simulink model "sampleModel7323_pp_1_1"  (R2018a)
settings: Solver=VariableStepAuto  StartTime=0.0  StopTime=10.0  RelTol=1e-3
undefined symbols (not defined in the file): DiscIntNeverNeededParam
libraries: simulink x65
(part 1 of 2)
settings Model: Creator=cyfuzz  LastModifiedBy=shafiul
settings CodeAppCC: StateflowObjectComments=on

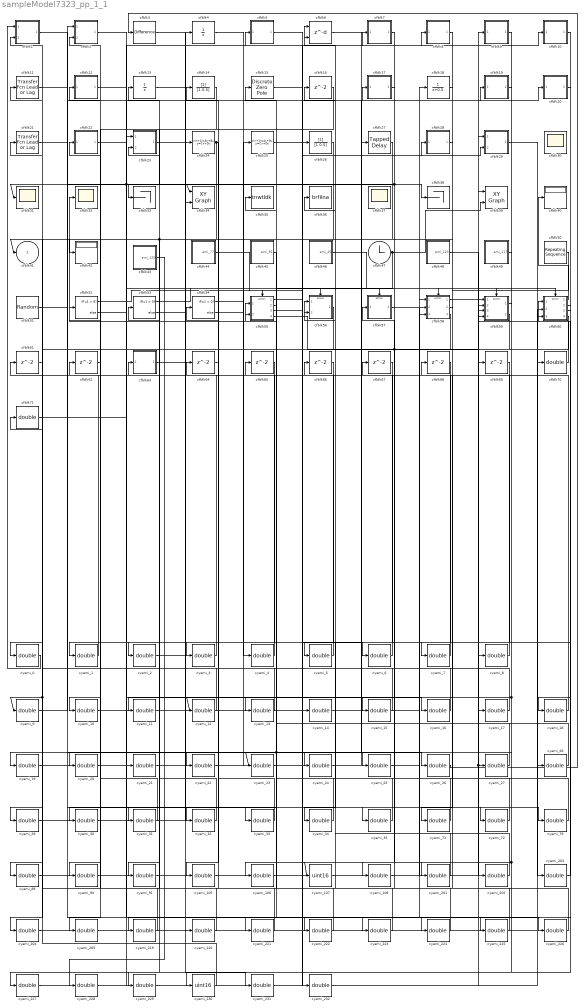
== system sampleModel7323_pp_1_1 ==
  cfblk1 : Subsystem  TreatAsAtomicUnit=on
  cfblk10 : Subsystem  TreatAsAtomicUnit=on
  cfblk11 : simulink/Discrete/Transfer Fcn Lead or Lag  PoleZ=0.95  ZeroZ=0.75  ICPrevOutput=0.0  ICPrevInput=0.0  DoSatur=off
      settings: SourceProductName=Simulink  SourceProductBaseCode=SL
  cfblk12 : Subsystem  TreatAsAtomicUnit=on
  cfblk13 : UnitDelay
  cfblk14 : DiscreteFilter  SampleTime=1
  cfblk15 : DiscreteZeroPole  Poles=[0 0.5]  Gain=1
  cfblk{16,61..62,64..69} (9 alike) : Delay  SampleTime=1
  cfblk17 : Subsystem  TreatAsAtomicUnit=on
  cfblk18 : DiscreteTransferFcn  SampleTime=1
  cfblk19 : Subsystem  TreatAsAtomicUnit=on
  cfblk2 : Subsystem  TreatAsAtomicUnit=on
  cfblk20 : Subsystem  TreatAsAtomicUnit=on
  cfblk21 : simulink/Discrete/Transfer Fcn Lead or Lag  PoleZ=0.95  ZeroZ=0.75  ICPrevOutput=0.0  ICPrevInput=0.0  DoSatur=off
      settings: SourceProductName=Simulink  SourceProductBaseCode=SL
  cfblk22 : Subsystem  TreatAsAtomicUnit=on
  cfblk23 : Subsystem  TreatAsAtomicUnit=on
  cfblk24 : DiscreteStateSpace
  cfblk25 : DiscreteStateSpace
  cfblk26 : DiscreteFilter  SampleTime=1
  cfblk27 : simulink/Discrete/Tapped Delay  vinit=0.0  samptime=-1  NumDelays=1  DelayOrder=Oldest  includeCurrent=off
  cfblk28 : Subsystem  TreatAsAtomicUnit=on
  cfblk29 : Subsystem  TreatAsAtomicUnit=on
  cfblk3 : simulink/Discrete/Difference  ICPrevInput=0.0  OutMin=[]  OutMax=[]  OutDataTypeStr=double  OutputDataTypeScalingMode=double  OutDataType=fixdt(1, 16)  OutScaling=2^-10  DoSatur=off
  cfblk{30..32,37} (4 alike) : Scope
      cfblk30 settings: Floating=on
      cfblk37 settings: Floating=on
  cfblk33 : Terminator
  cfblk34 : simulink/Sinks/XY Graph  xmin=-1  xmax=1  ymin=-1  ymax=1  st=-1
  cfblk35 : ToWorkspace  VariableName=tnwtldk  SaveFormat=Timeseries  SampleTime=-1
  cfblk36 : ToWorkspace  VariableName=brfiina  SaveFormat=Timeseries  SampleTime=-1
  cfblk38 : Terminator
  cfblk39 : simulink/Sinks/XY Graph  xmin=-1  xmax=1  ymin=-1  ymax=1  st=-1
  cfblk4 : UnitDelay
  cfblk40 : Display
  cfblk42 : Display
  cfblk43 : Subsystem  TreatAsAtomicUnit=on
  cfblk44 : Subsystem  TreatAsAtomicUnit=on
  cfblk45 : Subsystem  TreatAsAtomicUnit=on
  cfblk46 : Subsystem  TreatAsAtomicUnit=on
  cfblk47 : Clock
  cfblk48 : Subsystem  TreatAsAtomicUnit=on
  cfblk49 : Subsystem  TreatAsAtomicUnit=on
  cfblk5 : Subsystem  TreatAsAtomicUnit=on
  cfblk50 : simulink/Sources/Repeating Sequence  rep_seq_t=[0 2]  rep_seq_y=[0 2]
  cfblk51 : UniformRandomNumber  SampleTime=0.1
  cfblk52 : If  SampleTime=1
  cfblk53 : If  SampleTime=1
  cfblk54 : If  SampleTime=1
  cfblk55 : Subsystem  TreatAsAtomicUnit=on
  cfblk56 : Subsystem  TreatAsAtomicUnit=on
  cfblk57 : Subsystem  TreatAsAtomicUnit=on
  cfblk58 : Subsystem  TreatAsAtomicUnit=on
  cfblk59 : Subsystem  TreatAsAtomicUnit=on
  cfblk6 : Delay  DelayLengthSource=Input port  SampleTime=1
      settings: InputPortMap=u0,p1
  cfblk60 : Subsystem  TreatAsAtomicUnit=on
  cfblk63 : Subsystem  TreatAsAtomicUnit=on
  cfblk7 : Subsystem  TreatAsAtomicUnit=on
  cfblk70 : DataTypeConversion  OutDataTypeStr=double
  cfblk71 : DataTypeConversion  OutDataTypeStr=double
  cfblk8 : Subsystem  TreatAsAtomicUnit=on
  cfblk9 : Subsystem  TreatAsAtomicUnit=on
  cyemi_{0..35,71..72,79,89..91,105..106,108,201..205,219..229,231..232} (63 alike) : DataTypeConversion  OutDataTypeStr=double
  cyemi_107 : DataTypeConversion  OutDataTypeStr=uint16
  cyemi_230 : DataTypeConversion  OutDataTypeStr=uint16
  cfblk41 : Outport
  wires:
  cfblk55/2(cfblk13) -> cfblk32/1
  cfblk24/1 -> cfblk41/1, cyemi_91/1, cyemi_32/1
  cfblk56/1(cfblk2) -> cyemi_9/1, cyemi_204/1
  cfblk60/1(cfblk2) -> cfblk40/1
  cfblk11/1 -> cfblk38/1
  cfblk16/1 -> cfblk33/1
  cfblk47/1 -> cfblk39/2, cyemi_13/1
  cfblk60/4(cfblk16) -> cyemi_108/1, cyemi_221/1
  cfblk52/1 -> cfblk55/Action
  cfblk52/2 -> cfblk56/Action
  cfblk53/1 -> cfblk57/Action
  cfblk53/2 -> cfblk58/Action
  cfblk54/1 -> cfblk59/Action
  cfblk54/2 -> cfblk60/Action
  cfblk70/1 -> cfblk39/1
  cfblk61/1 -> cyemi_0/1
  cfblk67/1 -> cyemi_1/1
  cfblk60/2(cfblk14) -> cyemi_2/1
  cyemi_3/1 -> cfblk11/1
  cfblk4/1 -> cyemi_4/1
  cyemi_5/1 -> cfblk13/1
  cfblk58/2(cfblk16) -> cyemi_5/1
  cyemi_6/1 -> cfblk14/1
  cyemi_7/1 -> cfblk15/1
  cfblk59/2(cfblk16) -> cyemi_7/1
  cyemi_8/1 -> cfblk16/1
  cfblk55/4(cfblk15) -> cyemi_8/1
  cyemi_10/1 -> cfblk18/1
  cfblk14/1 -> cyemi_10/1
  cfblk59/1(cfblk2) -> cyemi_11/1
  cfblk55/3(cfblk14) -> cyemi_14/1
  cyemi_15/1 -> cfblk21/1
  cfblk13/1 -> cyemi_16/1
  cfblk58/1(cfblk2) -> cyemi_17/1
  cfblk60/3(cfblk15) -> cyemi_18/1
  cyemi_19/1 -> cfblk24/1
  cfblk50/1 -> cyemi_19/1
  cyemi_20/1 -> cfblk25/1
  cyemi_21/1 -> cfblk26/1
  cfblk71/1 -> cyemi_21/1
  cyemi_22/1 -> cfblk27/1
  cfblk51/1 -> cyemi_24/1
  cyemi_26/1 -> cfblk3/1
  cfblk6/1 -> cyemi_26/1
  cyemi_27/1 -> cfblk35/1
  cyemi_28/1 -> cfblk36/1
  cyemi_29/1 -> cfblk4/1
  cfblk58/3(cfblk17) -> cyemi_29/1
  cyemi_31/1 -> cfblk52/1
  cfblk66/1 -> cyemi_31/1
  cyemi_32/1 -> cfblk53/1
  cyemi_33/1 -> cfblk54/1
  cfblk68/1 -> cyemi_33/1
  cyemi_34/1 -> cfblk55/1(cfblk1)
  cfblk69/1 -> cyemi_34/1
  cyemi_35/1 -> cfblk55/2(cfblk12)
  cyemi_71/1 -> cfblk56/1(cfblk1)
  cfblk18/1 -> cyemi_71/1
  cyemi_72/1 -> cfblk56/2(cfblk7)
  cyemi_79/1 -> cfblk57/1(cfblk1)
  cfblk55/1(cfblk2) -> cyemi_79/1
  cyemi_89/1 -> cfblk58/1(cfblk1)
  cfblk27/1 -> cyemi_89/1
  cyemi_90/1 -> cfblk58/2(cfblk14)
  cfblk65/1 -> cyemi_90/1
  cyemi_91/1 -> cfblk58/3(cfblk15)
  cyemi_105/1 -> cfblk59/1(cfblk1)
  cfblk64/1 -> cyemi_105/1
  cyemi_106/1 -> cfblk59/2(cfblk13)
  cyemi_107/1 -> cfblk59/3(cfblk14)
  cyemi_108/1 -> cfblk59/4(cfblk15)
  cyemi_201/1 -> cfblk6/1
  cyemi_202/1 -> cfblk6/2
  cyemi_203/1 -> cfblk60/1(cfblk1)
  cyemi_204/1 -> cfblk60/2(cfblk12)
  cyemi_205/1 -> cfblk60/3(cfblk13)
  cfblk62/1 -> cyemi_205/1
  cyemi_219/1 -> cfblk61/1
  cyemi_220/1 -> cfblk62/1
  cyemi_222/1 -> cfblk64/1
  cyemi_223/1 -> cfblk65/1
  cfblk25/1 -> cyemi_223/1
  cyemi_224/1 -> cfblk66/1
  cyemi_225/1 -> cfblk67/1
  cfblk21/1 -> cyemi_225/1
  cyemi_226/1 -> cfblk68/1
  cfblk57/1(cfblk2) -> cyemi_226/1
  cyemi_227/1 -> cfblk69/1
  cyemi_229/1 -> cfblk70/1
  cfblk26/1 -> cyemi_229/1
  cyemi_230/1 -> cfblk71/1
  cfblk3/1 -> cyemi_231/1
  cfblk15/1 -> cyemi_232/1
  cyemi_221/1 -> cfblk63/1(emi_6)
  cfblk63/1(emi_7) -> cyemi_35/1
  cyemi_11/1 -> cfblk19/1(emi_9)
  cfblk19/1(emi_10) -> cyemi_201/1
  cyemi_228/1 -> cfblk7/1(emi_15)
  cfblk7/1(emi_16) -> cyemi_106/1, cfblk31/1
  cyemi_9/1 -> cfblk17/1(emi_30)
  cfblk17/1(emi_31) -> cyemi_22/1, cfblk34/1
  cyemi_4/1 -> cfblk12/1(emi_39)
  cfblk12/1(emi_40) -> cyemi_15/1
  cfblk46/1(emi_45) -> cyemi_28/1
  cyemi_24/1 -> cfblk29/1(emi_47)
  cyemi_25/1 -> cfblk29/2(emi_48)
  cfblk29/1(emi_49) -> cyemi_203/1
  cyemi_16/1 -> cfblk22/1(emi_54)
  cfblk22/1(emi_55) -> cyemi_224/1, cfblk34/2
  cyemi_23/1 -> cfblk28/1(emi_64)
  cfblk28/1(emi_65) -> cyemi_3/1
  cyemi_14/1 -> cfblk20/1(emi_67)
  cfblk20/1(emi_68) -> cyemi_227/1
  cyemi_17/1 -> cfblk23/1(emi_73)
  cyemi_18/1 -> cfblk23/2(emi_74)
  cfblk23/1(emi_75) -> cyemi_220/1
  cfblk44/1(emi_77) -> cyemi_6/1
  cyemi_30/1 -> cfblk5/1(emi_79)
  cfblk5/1(emi_80) -> cyemi_25/1
  cyemi_2/1 -> cfblk10/1(emi_82)
  cfblk10/1(emi_83) -> cyemi_219/1
  cyemi_231/1 -> cfblk8/1(emi_85)
  cfblk8/1(emi_86) -> cfblk42/1
  cfblk45/1(emi_91) -> cyemi_30/1, cyemi_23/1
  cyemi_12/1 -> cfblk2/1(emi_103)
  cyemi_13/1 -> cfblk2/2(emi_104)
  cfblk2/1(emi_105) -> cyemi_222/1
  cyemi_232/1 -> cfblk9/1(emi_107)
  cfblk9/1(emi_108) -> cyemi_20/1, cyemi_12/1
  cyemi_0/1 -> cfblk1/1(emi_113)
  cyemi_1/1 -> cfblk1/2(emi_114)
  cfblk1/1(emi_115) -> cyemi_72/1
  cfblk49/1(emi_117) -> cyemi_107/1, cyemi_230/1
  cfblk48/1(emi_123) -> cyemi_202/1, cyemi_27/1
  cfblk43/1(emi_125) -> cyemi_228/1

== system sampleModel7323_pp_1_1/cfblk1 ==
  emi_113 : Inport  Partition=on  PartitionDimension=1  PartitionWidth=1  PartitionOffset=0
  emi_114 : Inport  Port=2  Partition=on  PartitionDimension=1  PartitionWidth=1  PartitionOffset=0
  For Each : ForEach  DisableCoverage=on  IndexMode=One-based
  cfblk1 : Delay  ShowEnablePort=on  SampleTime=1
      settings: InputPortMap=u0,e6
  emi_115 : Outport  ConcatenationDimension=1
  wires:
  emi_113/1 -> cfblk1/1
  emi_114/1 -> cfblk1/2
  cfblk1/1 -> emi_115/1

== system sampleModel7323_pp_1_1/cfblk10 ==
  emi_82 : Inport  Partition=on  PartitionDimension=1  PartitionWidth=1  PartitionOffset=0
  For Each : ForEach  DisableCoverage=on  IndexMode=One-based
  cfblk10 : simulink/Discrete/Difference  ICPrevInput=0.0  OutMin=[]  OutMax=[]  OutDataTypeStr=double  OutputDataTypeScalingMode=double  OutDataType=fixdt(1, 16)  OutScaling=2^-10  DoSatur=off
  emi_83 : Outport  ConcatenationDimension=1
  wires:
  emi_82/1 -> cfblk10/1
  cfblk10/1 -> emi_83/1

== system sampleModel7323_pp_1_1/cfblk12 ==
  emi_39 : Inport  Partition=on  PartitionDimension=1  PartitionWidth=1  PartitionOffset=0
  For Each : ForEach  DisableCoverage=on  IndexMode=One-based
  cfblk12 : DiscreteFilter  SampleTime=1
  emi_40 : Outport  ConcatenationDimension=1
  wires:
  emi_39/1 -> cfblk12/1
  cfblk12/1 -> emi_40/1

== system sampleModel7323_pp_1_1/cfblk17 ==
  emi_30 : Inport  Partition=on  PartitionDimension=1  PartitionWidth=1  PartitionOffset=0
  For Each : ForEach  DisableCoverage=on  IndexMode=One-based
  cfblk17 : simulink/Discrete/Tapped Delay  vinit=0.0  samptime=-1  NumDelays=1  DelayOrder=Oldest  includeCurrent=off
  emi_31 : Outport  ConcatenationDimension=1
  wires:
  emi_30/1 -> cfblk17/1
  cfblk17/1 -> emi_31/1

== system sampleModel7323_pp_1_1/cfblk19 ==
  emi_9 : Inport  Partition=on  PartitionDimension=1  PartitionWidth=1  PartitionOffset=0
  For Each : ForEach  DisableCoverage=on  IndexMode=One-based
  cfblk19 : simulink/Discrete/Difference  ICPrevInput=0.0  OutMin=[]  OutMax=[]  OutDataTypeStr=double  OutputDataTypeScalingMode=double  OutDataType=fixdt(1, 16)  OutScaling=2^-10  DoSatur=off
  emi_10 : Outport  ConcatenationDimension=1
  wires:
  emi_9/1 -> cfblk19/1
  cfblk19/1 -> emi_10/1

== system sampleModel7323_pp_1_1/cfblk2 ==
  emi_103 : Inport  Partition=on  PartitionDimension=1  PartitionWidth=1  PartitionOffset=0
  emi_104 : Inport  Port=2  Partition=on  PartitionDimension=1  PartitionWidth=1  PartitionOffset=0
  For Each : ForEach  DisableCoverage=on  IndexMode=One-based
  cfblk2 : Delay  ShowEnablePort=on  SampleTime=1
      settings: InputPortMap=u0,e6
  emi_105 : Outport  ConcatenationDimension=1
  wires:
  emi_103/1 -> cfblk2/1
  emi_104/1 -> cfblk2/2
  cfblk2/1 -> emi_105/1

== system sampleModel7323_pp_1_1/cfblk20 ==
  emi_67 : Inport  Partition=on  PartitionDimension=1  PartitionWidth=1  PartitionOffset=0
  For Each : ForEach  DisableCoverage=on  IndexMode=One-based
  cfblk20 : Subsystem  TreatAsAtomicUnit=on
  emi_68 : Outport  ConcatenationDimension=1
  wires:
  emi_67/1 -> cfblk20/1(emi_33)
  cfblk20/1(emi_34) -> emi_68/1

== system sampleModel7323_pp_1_1/cfblk22 ==
  emi_54 : Inport  Partition=on  PartitionDimension=1  PartitionWidth=1  PartitionOffset=0
  For Each : ForEach  DisableCoverage=on  IndexMode=One-based
  cfblk22 : simulink/Continuous/PID Controller  Controller=PID  TimeDomain=Discrete-time  SampleTime=1  IntegratorMethod=Forward Euler  FilterMethod=Forward Euler  Form=Parallel  UseFilter=on  ControllerParametersSource=internal  P=1  I=1  D=0  N=100  InitialConditionSource=internal  InitialConditionForIntegrator=0  InitialConditionForFilter=0  ExternalReset=none  LimitOutput=off  UpperSaturationLimit=inf  LowerSaturationLimit=-inf  LinearizeAsGain=off  AntiWindupMode=none  Kb=1  TrackingMode=off  Kt=1  PParamMin=[]  PParamMax=[]  IParamMin=[]  IParamMax=[]  DParamMin=[]  DParamMax=[]  NParamMin=[]  NParamMax=[]  KbParamMin=[]  KbParamMax=[]  KtParamMin=[]  KtParamMax=[]  POutMin=[]  POutMax=[]  IOutMin=[]  IOutMax=[]  DOutMin=[]  DOutMax=[]  NOutMin=[]  NOutMax=[]  KbOutMin=[]  KbOutMax=[]  KtOutMin=[]  KtOutMax=[]  IntegratorOutMin=[]  IntegratorOutMax=[]  FilterOutMin=[]  FilterOutMax=[]  SumOutMin=[]  SumOutMax=[]  SumI1OutMin=[]  SumI1OutMax=[]  SumI2OutMin=[]  SumI2OutMax=[]  SumI3OutMin=[]  SumI3OutMax=[]  SumDOutMin=[]  SumDOutMax=[]  SaturationOutMin=[]  SaturationOutMax=[]  IntegratorContinuousStateAttributes=''  IntegratorStateMustResolveToSignalObject=off  IntegratorRTWStateStorageClass=Auto  FilterContinuousStateAttributes=''  FilterStateMustResolveToSignalObject=off  FilterRTWStateStorageClass=Auto  DifferentiatorICPrevScaledInput=0  DifferentiatorOutMin=[]  DifferentiatorOutMax=[]  FilterDiffOutCoefMin=[]  FilterDiffOutCoefMax=[]  SumDenOutMin=[]  SumDenOutMax=[]  SumNumOutMin=[]  SumNumOutMax=[]  ReciprocalOutMin=[]  ReciprocalOutMax=[]  DivideOutMin=[]  DivideOutMax=[]  TunerSelectOption=Transfer Function Based (PID Tuner App)
  emi_55 : Outport  ConcatenationDimension=1
  wires:
  emi_54/1 -> cfblk22/1
  cfblk22/1 -> emi_55/1

== system sampleModel7323_pp_1_1/cfblk23 ==
  emi_73 : Inport  Partition=on  PartitionDimension=1  PartitionWidth=1  PartitionOffset=0
  emi_74 : Inport  Port=2  Partition=on  PartitionDimension=1  PartitionWidth=1  PartitionOffset=0
  For Each : ForEach  DisableCoverage=on  IndexMode=One-based
  cfblk23 : Subsystem  TreatAsAtomicUnit=on
  emi_75 : Outport  ConcatenationDimension=1
  wires:
  emi_73/1 -> cfblk23/1(emi_60)
  emi_74/1 -> cfblk23/2(emi_61)
  cfblk23/1(emi_62) -> emi_75/1

== system sampleModel7323_pp_1_1/cfblk28 ==
  emi_64 : Inport  Partition=on  PartitionDimension=1  PartitionWidth=1  PartitionOffset=0
  For Each : ForEach  DisableCoverage=on  IndexMode=One-based
  cfblk28 : simulink/Discrete/Difference  ICPrevInput=0.0  OutMin=[]  OutMax=[]  OutDataTypeStr=double  OutputDataTypeScalingMode=double  OutDataType=fixdt(1, 16)  OutScaling=2^-10  DoSatur=off
  emi_65 : Outport  ConcatenationDimension=1
  wires:
  emi_64/1 -> cfblk28/1
  cfblk28/1 -> emi_65/1

== system sampleModel7323_pp_1_1/cfblk29 ==
  emi_47 : Inport  Partition=on  PartitionDimension=1  PartitionWidth=1  PartitionOffset=0
  emi_48 : Inport  Port=2  Partition=on  PartitionDimension=1  PartitionWidth=1  PartitionOffset=0
  For Each : ForEach  DisableCoverage=on  IndexMode=One-based
  cfblk29 : simulink/Continuous/PID Controller (2DOF)  Controller=PID  TimeDomain=Discrete-time  SampleTime=1  IntegratorMethod=Forward Euler  FilterMethod=Forward Euler  Form=Parallel  UseFilter=on  ControllerParametersSource=internal  P=1  I=1  D=0  N=100  b=1  c=1  InitialConditionSource=internal  InitialConditionForIntegrator=0  InitialConditionForFilter=0  ExternalReset=none  LimitOutput=off  UpperSaturationLimit=inf  LowerSaturationLimit=-inf  LinearizeAsGain=off  AntiWindupMode=none  Kb=1  TrackingMode=off  Kt=1  PParamMin=[]  PParamMax=[]  IParamMin=[]  IParamMax=[]  DParamMin=[]  DParamMax=[]  NParamMin=[]  NParamMax=[]  bParamMin=[]  bParamMax=[]  cParamMin=[]  cParamMax=[]  KbParamMin=[]  KbParamMax=[]  KtParamMin=[]  KtParamMax=[]  POutMin=[]  POutMax=[]  IOutMin=[]  IOutMax=[]  DOutMin=[]  DOutMax=[]  NOutMin=[]  NOutMax=[]  bOutMin=[]  bOutMax=[]  cOutMin=[]  cOutMax=[]  KbOutMin=[]  KbOutMax=[]  KtOutMin=[]  KtOutMax=[]  IntegratorOutMin=[]  IntegratorOutMax=[]  FilterOutMin=[]  FilterOutMax=[]  SumOutMin=[]  SumOutMax=[]  Sum1OutMin=[]  Sum1OutMax=[]  Sum2OutMin=[]  Sum2OutMax=[]  Sum3OutMin=[]  Sum3OutMax=[]  SumI1OutMin=[]  SumI1OutMax=[]  SumI2OutMin=[]  SumI2OutMax=[]  SumI3OutMin=[]  SumI3OutMax=[]  SumDOutMin=[]  SumDOutMax=[]  SaturationOutMin=[]  SaturationOutMax=[]  IntegratorContinuousStateAttributes=''  IntegratorStateMustResolveToSignalObject=off  IntegratorRTWStateStorageClass=Auto  FilterContinuousStateAttributes=''  FilterStateMustResolveToSignalObject=off  FilterRTWStateStorageClass=Auto  DifferentiatorICPrevScaledInput=0  DifferentiatorOutMin=[]  DifferentiatorOutMax=[]  FilterDiffOutCoefMin=[]  FilterDiffOutCoefMax=[]  SumDenOutMin=[]  SumDenOutMax=[]  SumNumOutMin=[]  SumNumOutMax=[]  ReciprocalOutMin=[]  ReciprocalOutMax=[]  DivideOutMin=[]  DivideOutMax=[]  TunerSelectOption=Transfer Function Based (PID Tuner App)
  emi_49 : Outport  ConcatenationDimension=1
  wires:
  emi_47/1 -> cfblk29/1
  emi_48/1 -> cfblk29/2
  cfblk29/1 -> emi_49/1

== system sampleModel7323_pp_1_1/cfblk43 ==
  For Each : ForEach  DisableCoverage=on  IndexMode=One-based
  cfblk43 : simulink/Sources/Chirp Signal  f1=0.1  T=100  f2=1
  emi_125 : Outport  ConcatenationDimension=1
  wires:
  cfblk43/1 -> emi_125/1

== system sampleModel7323_pp_1_1/cfblk44 ==
  For Each : ForEach  DisableCoverage=on  IndexMode=One-based
  cfblk44 : Constant  Value=0797  OutDataTypeStr=double  SampleTime=1
  emi_77 : Outport  ConcatenationDimension=1
  wires:
  cfblk44/1 -> emi_77/1

== system sampleModel7323_pp_1_1/cfblk45 ==
  For Each : ForEach  DisableCoverage=on  IndexMode=One-based
  cfblk45 : simulink/Sources/Repeating Sequence Stair  OutValues=[3 1 4 2 1].'  tsamp=1  OutMin=[]  OutMax=[]  OutDataTypeStr=double  OutputDataTypeScalingMode=double  OutDataType=fixdt(0,8)  ConRadixGroup=Best Precision: Vector-wise  OutScaling=2^-12
  emi_91 : Outport  ConcatenationDimension=1
  wires:
  cfblk45/1 -> emi_91/1

== system sampleModel7323_pp_1_1/cfblk46 ==
  For Each : ForEach  DisableCoverage=on  IndexMode=One-based
  cfblk46 : simulink/Sources/Chirp Signal  f1=0.1  T=100  f2=1
  emi_45 : Outport  ConcatenationDimension=1
  wires:
  cfblk46/1 -> emi_45/1

== system sampleModel7323_pp_1_1/cfblk48 ==
  For Each : ForEach  DisableCoverage=on  IndexMode=One-based
  cfblk48 : DiscretePulseGenerator  PulseType=Time based  Period=10  PulseWidth=5
  emi_123 : Outport  ConcatenationDimension=1
  wires:
  cfblk48/1 -> emi_123/1

== system sampleModel7323_pp_1_1/cfblk49 ==
  For Each : ForEach  DisableCoverage=on  IndexMode=One-based
  cfblk49 : Subsystem  TreatAsAtomicUnit=on
  emi_117 : Outport  ConcatenationDimension=1
  wires:
  cfblk49/1(emi_4) -> emi_117/1

== system sampleModel7323_pp_1_1/cfblk5 ==
  emi_79 : Inport  Partition=on  PartitionDimension=1  PartitionWidth=1  PartitionOffset=0
  For Each : ForEach  DisableCoverage=on  IndexMode=One-based
  cfblk5 : simulink/Discrete/Transfer Fcn Real Zero  ZeroZ=0.75  ICPrevInput=0.0  DoSatur=off
      settings: SourceProductName=Simulink  SourceProductBaseCode=SL
  emi_80 : Outport  ConcatenationDimension=1
  wires:
  emi_79/1 -> cfblk5/1
  cfblk5/1 -> emi_80/1

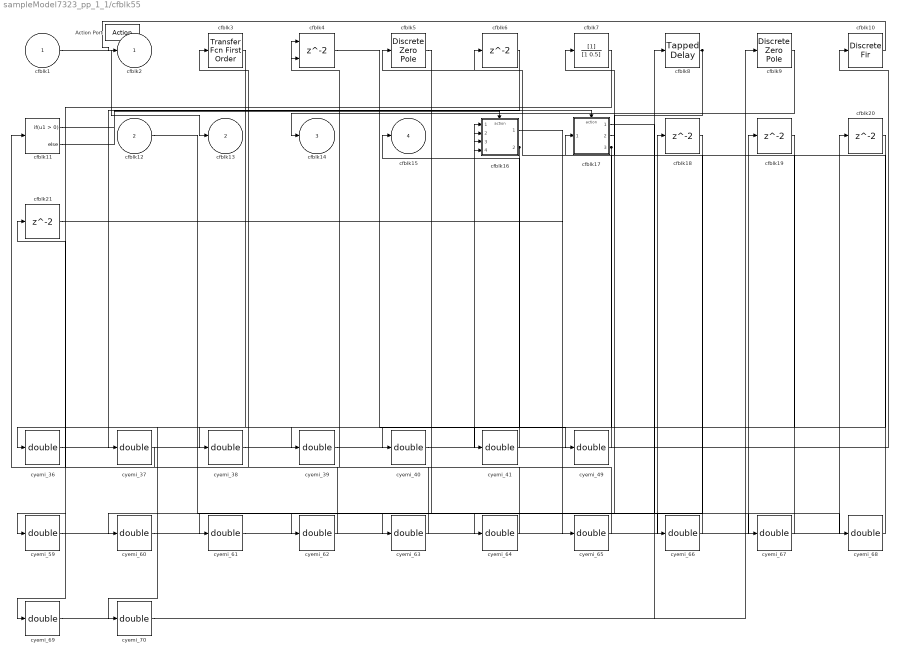
== system sampleModel7323_pp_1_1/cfblk55 ==
  cfblk1 : Inport
  cfblk12 : Inport  Port=2
  Action Port : ActionPort  ActionType=then
  cfblk10 : DiscreteFir
  cfblk11 : If  SampleTime=1
  cfblk16 : Subsystem  TreatAsAtomicUnit=on
  cfblk17 : Subsystem  TreatAsAtomicUnit=on
  cfblk{6,18..21} (5 alike) : Delay
  cfblk3 : simulink/Discrete/Transfer Fcn First Order  PoleZ=0.95  ICPrevOutput=0.0  DoSatur=off
      settings: SourceProductName=Simulink
  cfblk4 : Delay  ShowEnablePort=on
      settings: InputPortMap=u0,e6
  cfblk5 : DiscreteZeroPole  Poles=[0 0.5]  Gain=1  SampleTime=-1
  cfblk7 : DiscreteFilter
  cfblk8 : simulink/Discrete/Tapped Delay  vinit=0.0  samptime=-1  NumDelays=1  DelayOrder=Oldest  includeCurrent=off
  cfblk9 : DiscreteZeroPole  Poles=[0 0.5]  Gain=1  SampleTime=-1
  cyemi_{36..41,49,59..70} (19 alike) : DataTypeConversion  OutDataTypeStr=double
  cfblk2 : Outport
  cfblk13 : Outport  Port=2
  cfblk14 : Outport  Port=3
  cfblk15 : Outport  Port=4
  wires:
  cfblk1/1 -> cfblk13/1
  cfblk10/1 -> cfblk2/1
  cfblk8/1 -> cyemi_60/1, cyemi_61/1, cyemi_62/1
  cfblk9/1 -> cfblk14/1
  cfblk17/3(cfblk11) -> cyemi_40/1, cyemi_69/1
  cfblk16/2(cfblk12) -> cfblk15/1, cyemi_59/1
  cfblk11/1 -> cfblk16/Action
  cfblk11/2 -> cfblk17/Action
  cyemi_36/1 -> cfblk10/1
  cfblk7/1 -> cyemi_36/1
  cyemi_37/1 -> cfblk11/1
  cfblk6/1 -> cyemi_37/1
  cyemi_38/1 -> cfblk16/1(cfblk1)
  cfblk19/1 -> cyemi_38/1
  cyemi_39/1 -> cfblk16/2(cfblk9)
  cfblk17/2(cfblk10) -> cyemi_39/1
  cyemi_40/1 -> cfblk16/3(cfblk10)
  cyemi_41/1 -> cfblk16/4(cfblk11)
  cfblk20/1 -> cyemi_41/1
  cyemi_49/1 -> cfblk17/1(cfblk1)
  cfblk4/1 -> cyemi_49/1
  cyemi_59/1 -> cfblk18/1
  cyemi_60/1 -> cfblk19/1
  cyemi_61/1 -> cfblk20/1
  cyemi_62/1 -> cfblk21/1
  cyemi_63/1 -> cfblk3/1
  cfblk5/1 -> cyemi_63/1
  cyemi_64/1 -> cfblk4/1
  cfblk18/1 -> cyemi_64/1
  cyemi_65/1 -> cfblk4/2
  cfblk21/1 -> cyemi_65/1
  cyemi_66/1 -> cfblk5/1
  cfblk16/1(cfblk2) -> cyemi_66/1
  cyemi_67/1 -> cfblk6/1
  cfblk12/1 -> cyemi_67/1
  cyemi_68/1 -> cfblk7/1
  cfblk17/1(cfblk2) -> cyemi_68/1
  cyemi_69/1 -> cfblk8/1
  cyemi_70/1 -> cfblk9/1
  cfblk3/1 -> cyemi_70/1

== system sampleModel7323_pp_1_1/cfblk56 ==
  cfblk1 : Inport
  cfblk7 : Inport  Port=2
  Action Port : ActionPort  ActionType=else
  cfblk3 : Subsystem  TreatAsAtomicUnit=on
  cfblk4 : Delay  ShowEnablePort=on
      settings: InputPortMap=u0,e6
  cfblk5 : Subsystem  TreatAsAtomicUnit=on
  cfblk6 : Subsystem  TreatAsAtomicUnit=on
  cfblk8 : Delay
  cyemi_{73..78} (6 alike) : DataTypeConversion  OutDataTypeStr=double
  cfblk2 : Outport
  wires:
  cfblk8/1 -> cyemi_73/1
  cyemi_74/1 -> cfblk4/1
  cfblk7/1 -> cyemi_74/1
  cyemi_75/1 -> cfblk4/2
  cfblk1/1 -> cyemi_75/1
  cfblk4/1 -> cyemi_77/1
  cyemi_78/1 -> cfblk8/1
  cyemi_77/1 -> cfblk6/1(emi_1)
  cfblk6/1(emi_2) -> cfblk2/1
  cyemi_76/1 -> cfblk5/1(emi_21)
  cfblk5/1(emi_22) -> cyemi_78/1
  cyemi_73/1 -> cfblk3/1(emi_110)
  cfblk3/1(emi_111) -> cyemi_76/1

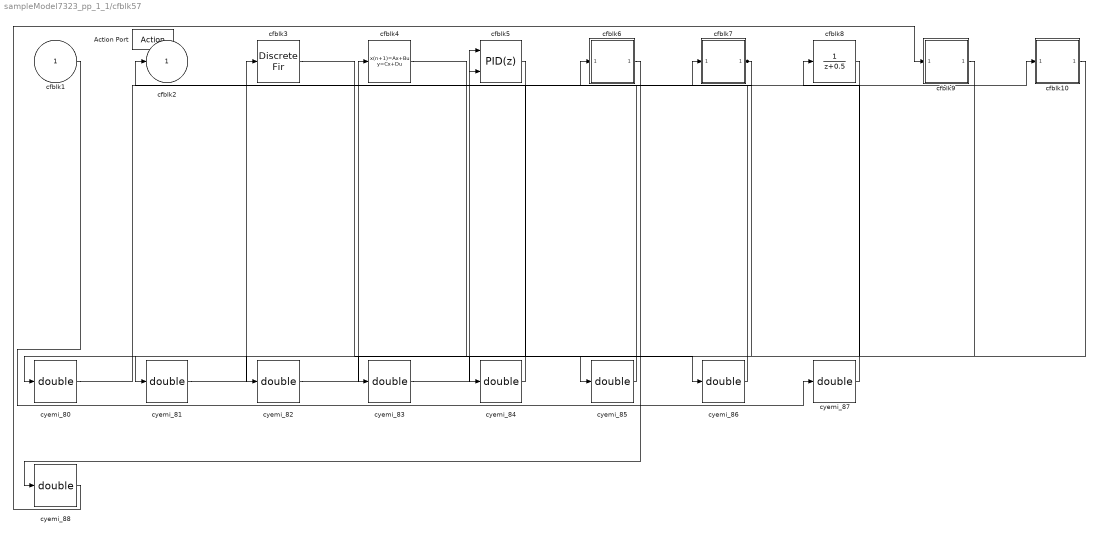
== system sampleModel7323_pp_1_1/cfblk57 ==
  cfblk1 : Inport
  Action Port : ActionPort  ActionType=then
  cfblk10 : Subsystem  TreatAsAtomicUnit=on
  cfblk3 : DiscreteFir
  cfblk4 : DiscreteStateSpace  SampleTime=-1
  cfblk5 : simulink/Continuous/PID Controller (2DOF)  Controller=PID  TimeDomain=Discrete-time  SampleTime=-1  IntegratorMethod=Forward Euler  FilterMethod=Forward Euler  Form=Parallel  UseFilter=on  ControllerParametersSource=internal  P=1  I=1  D=0  N=100  b=1  c=1  InitialConditionSource=internal  InitialConditionForIntegrator=0  InitialConditionForFilter=0  ExternalReset=none  LimitOutput=off  UpperSaturationLimit=inf  LowerSaturationLimit=-inf  LinearizeAsGain=off  AntiWindupMode=none  Kb=1  TrackingMode=off  Kt=1  PParamMin=[]  PParamMax=[]  IParamMin=[]  IParamMax=[]  DParamMin=[]  DParamMax=[]  NParamMin=[]  NParamMax=[]  bParamMin=[]  bParamMax=[]  cParamMin=[]  cParamMax=[]  KbParamMin=[]  KbParamMax=[]  KtParamMin=[]  KtParamMax=[]  POutMin=[]  POutMax=[]  IOutMin=[]  IOutMax=[]  DOutMin=[]  DOutMax=[]  NOutMin=[]  NOutMax=[]  bOutMin=[]  bOutMax=[]  cOutMin=[]  cOutMax=[]  KbOutMin=[]  KbOutMax=[]  KtOutMin=[]  KtOutMax=[]  IntegratorOutMin=[]  IntegratorOutMax=[]  FilterOutMin=[]  FilterOutMax=[]  SumOutMin=[]  SumOutMax=[]  Sum1OutMin=[]  Sum1OutMax=[]  Sum2OutMin=[]  Sum2OutMax=[]  Sum3OutMin=[]  Sum3OutMax=[]  SumI1OutMin=[]  SumI1OutMax=[]  SumI2OutMin=[]  SumI2OutMax=[]  SumI3OutMin=[]  SumI3OutMax=[]  SumDOutMin=[]  SumDOutMax=[]  SaturationOutMin=[]  SaturationOutMax=[]  IntegratorContinuousStateAttributes=''  IntegratorStateMustResolveToSignalObject=off  IntegratorRTWStateStorageClass=Auto  FilterContinuousStateAttributes=''  FilterStateMustResolveToSignalObject=off  FilterRTWStateStorageClass=Auto  DifferentiatorICPrevScaledInput=0  DifferentiatorOutMin=[]  DifferentiatorOutMax=[]  FilterDiffOutCoefMin=[]  FilterDiffOutCoefMax=[]  SumDenOutMin=[]  SumDenOutMax=[]  SumNumOutMin=[]  SumNumOutMax=[]  ReciprocalOutMin=[]  ReciprocalOutMax=[]  DivideOutMin=[]  DivideOutMax=[]  TunerSelectOption=Transfer Function Based (PID Tuner App)
  cfblk6 : Subsystem  TreatAsAtomicUnit=on
  cfblk7 : Subsystem  TreatAsAtomicUnit=on
  cfblk8 : DiscreteTransferFcn
  cfblk9 : Subsystem  TreatAsAtomicUnit=on
  cyemi_{80..88} (9 alike) : DataTypeConversion  OutDataTypeStr=double
  cfblk2 : Outport
  wires:
  cyemi_81/1 -> cfblk3/1
  cfblk5/1 -> cyemi_81/1
  cyemi_82/1 -> cfblk4/1
  cfblk8/1 -> cyemi_82/1
  cyemi_83/1 -> cfblk5/1
  cyemi_84/1 -> cfblk5/2
  cfblk4/1 -> cyemi_85/1
  cfblk3/1 -> cyemi_86/1
  cyemi_87/1 -> cfblk8/1
  cfblk1/1 -> cyemi_87/1
  cyemi_85/1 -> cfblk6/1(emi_24)
  cfblk6/1(emi_25) -> cyemi_88/1
  cyemi_88/1 -> cfblk9/1(emi_42)
  cfblk9/1(emi_43) -> cyemi_83/1
  cyemi_80/1 -> cfblk10/1(emi_57)
  cfblk10/1(emi_58) -> cyemi_84/1
  cyemi_86/1 -> cfblk7/1(emi_97)
  cfblk7/1(emi_98) -> cyemi_80/1, cfblk2/1

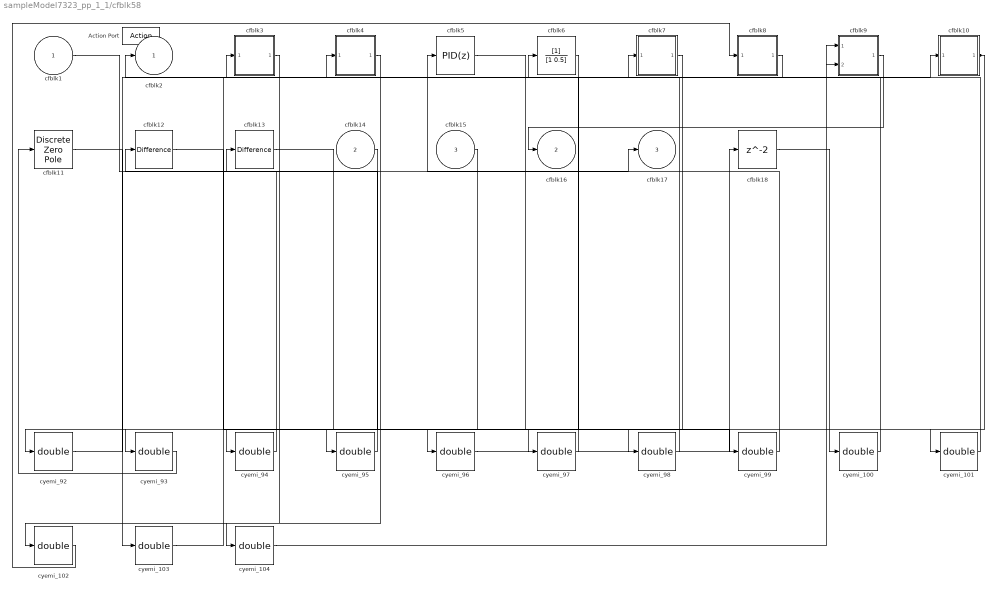
== system sampleModel7323_pp_1_1/cfblk58 ==
  cfblk1 : Inport
  cfblk14 : Inport  Port=2
  cfblk15 : Inport  Port=3
  Action Port : ActionPort  ActionType=else
  cfblk10 : Subsystem  TreatAsAtomicUnit=on
  cfblk11 : DiscreteZeroPole  Poles=[0 0.5]  Gain=1  SampleTime=-1
  cfblk12 : simulink/Discrete/Difference  ICPrevInput=0.0  OutMin=[]  OutMax=[]  OutDataTypeStr=double  OutputDataTypeScalingMode=double  OutDataType=fixdt(1, 16)  OutScaling=2^-10  DoSatur=off
  cfblk13 : simulink/Discrete/Difference  ICPrevInput=0.0  OutMin=[]  OutMax=[]  OutDataTypeStr=double  OutputDataTypeScalingMode=double  OutDataType=fixdt(1, 16)  OutScaling=2^-10  DoSatur=off
  cfblk18 : Delay
  cfblk3 : Subsystem  TreatAsAtomicUnit=on
  cfblk4 : Subsystem  TreatAsAtomicUnit=on
  cfblk5 : simulink/Continuous/PID Controller  Controller=PID  TimeDomain=Discrete-time  SampleTime=-1  IntegratorMethod=Forward Euler  FilterMethod=Forward Euler  Form=Parallel  UseFilter=on  ControllerParametersSource=internal  P=1  I=1  D=0  N=100  InitialConditionSource=internal  InitialConditionForIntegrator=0  InitialConditionForFilter=0  ExternalReset=none  LimitOutput=off  UpperSaturationLimit=inf  LowerSaturationLimit=-inf  LinearizeAsGain=off  AntiWindupMode=none  Kb=1  TrackingMode=off  Kt=1  PParamMin=[]  PParamMax=[]  IParamMin=[]  IParamMax=[]  DParamMin=[]  DParamMax=[]  NParamMin=[]  NParamMax=[]  KbParamMin=[]  KbParamMax=[]  KtParamMin=[]  KtParamMax=[]  POutMin=[]  POutMax=[]  IOutMin=[]  IOutMax=[]  DOutMin=[]  DOutMax=[]  NOutMin=[]  NOutMax=[]  KbOutMin=[]  KbOutMax=[]  KtOutMin=[]  KtOutMax=[]  IntegratorOutMin=[]  IntegratorOutMax=[]  FilterOutMin=[]  FilterOutMax=[]  SumOutMin=[]  SumOutMax=[]  SumI1OutMin=[]  SumI1OutMax=[]  SumI2OutMin=[]  SumI2OutMax=[]  SumI3OutMin=[]  SumI3OutMax=[]  SumDOutMin=[]  SumDOutMax=[]  SaturationOutMin=[]  SaturationOutMax=[]  IntegratorContinuousStateAttributes=''  IntegratorStateMustResolveToSignalObject=off  IntegratorRTWStateStorageClass=Auto  FilterContinuousStateAttributes=''  FilterStateMustResolveToSignalObject=off  FilterRTWStateStorageClass=Auto  DifferentiatorICPrevScaledInput=0  DifferentiatorOutMin=[]  DifferentiatorOutMax=[]  FilterDiffOutCoefMin=[]  FilterDiffOutCoefMax=[]  SumDenOutMin=[]  SumDenOutMax=[]  SumNumOutMin=[]  SumNumOutMax=[]  ReciprocalOutMin=[]  ReciprocalOutMax=[]  DivideOutMin=[]  DivideOutMax=[]  TunerSelectOption=Transfer Function Based (PID Tuner App)
  cfblk6 : DiscreteFilter
  cfblk7 : Subsystem  TreatAsAtomicUnit=on
  cfblk8 : Subsystem  TreatAsAtomicUnit=on
  cfblk9 : Subsystem  TreatAsAtomicUnit=on
  cyemi_{92..104} (13 alike) : DataTypeConversion  OutDataTypeStr=double
  cfblk2 : Outport
  cfblk16 : Outport  Port=2
  cfblk17 : Outport  Port=3
  wires:
  cfblk1/1 -> cfblk17/1
  cfblk6/1 -> cyemi_92/1
  cyemi_93/1 -> cfblk11/1
  cyemi_94/1 -> cfblk12/1
  cfblk15/1 -> cyemi_94/1
  cyemi_95/1 -> cfblk13/1
  cyemi_96/1 -> cfblk18/1
  cfblk13/1 -> cyemi_97/1
  cfblk5/1 -> cyemi_98/1
  cyemi_99/1 -> cfblk5/1
  cfblk12/1 -> cyemi_99/1
  cyemi_100/1 -> cfblk6/1
  cfblk18/1 -> cyemi_100/1
  cfblk11/1 -> cyemi_103/1
  cfblk14/1 -> cyemi_104/1
  cyemi_92/1 -> cfblk10/1(emi_12)
  cfblk10/1(emi_13) -> cyemi_101/1, cyemi_95/1
  cyemi_97/1 -> cfblk3/1(emi_27)
  cfblk3/1(emi_28) -> cyemi_93/1
  cyemi_101/1 -> cfblk7/1(emi_36)
  cfblk7/1(emi_37) -> cyemi_96/1
  cyemi_102/1 -> cfblk8/1(emi_70)
  cfblk8/1(emi_71) -> cfblk2/1
  cyemi_98/1 -> cfblk4/1(emi_88)
  cfblk4/1(emi_89) -> cyemi_102/1
  cyemi_103/1 -> cfblk9/1(emi_93)
  cyemi_104/1 -> cfblk9/2(emi_94)
  cfblk9/1(emi_95) -> cfblk16/1

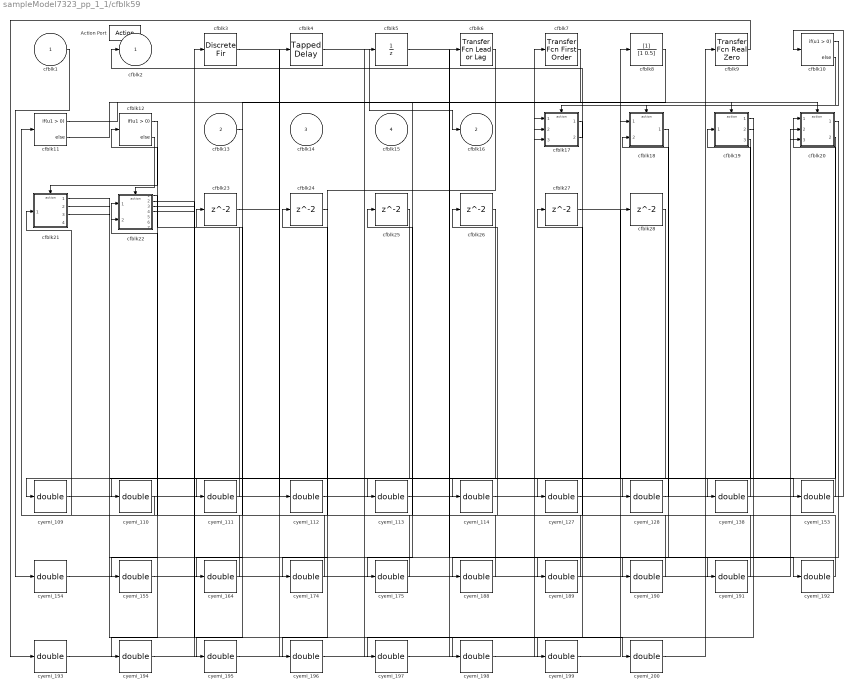
== system sampleModel7323_pp_1_1/cfblk59 ==
  cfblk1 : Inport
  cfblk13 : Inport  Port=2
  cfblk14 : Inport  Port=3
  cfblk15 : Inport  Port=4
  Action Port : ActionPort  ActionType=then
  cfblk10 : If  SampleTime=1
  cfblk11 : If  SampleTime=1
  cfblk12 : If  SampleTime=1
  cfblk17 : Subsystem  TreatAsAtomicUnit=on
  cfblk18 : Subsystem  TreatAsAtomicUnit=on
  cfblk19 : Subsystem  TreatAsAtomicUnit=on
  cfblk20 : Subsystem  TreatAsAtomicUnit=on
  cfblk21 : Subsystem  TreatAsAtomicUnit=on
  cfblk22 : Subsystem  TreatAsAtomicUnit=on
  cfblk{23..28} (6 alike) : Delay
  cfblk3 : DiscreteFir
  cfblk4 : simulink/Discrete/Tapped Delay  vinit=0.0  samptime=-1  NumDelays=1  DelayOrder=Oldest  includeCurrent=off
  cfblk5 : UnitDelay  SampleTime=-1
  cfblk6 : simulink/Discrete/Transfer Fcn Lead or Lag  PoleZ=0.95  ZeroZ=0.75  ICPrevOutput=0.0  ICPrevInput=0.0  DoSatur=off
      settings: SourceProductName=Simulink  SourceProductBaseCode=SL
  cfblk7 : simulink/Discrete/Transfer Fcn First Order  PoleZ=0.95  ICPrevOutput=0.0  DoSatur=off
      settings: SourceProductName=Simulink
  cfblk8 : DiscreteFilter
  cfblk9 : simulink/Discrete/Transfer Fcn Real Zero  ZeroZ=0.75  ICPrevInput=0.0  DoSatur=off
      settings: SourceProductName=Simulink  SourceProductBaseCode=SL
  cyemi_{109..114,127..128,138,153..155,164,174..175,188..200} (28 alike) : DataTypeConversion  OutDataTypeStr=double
  cfblk2 : Outport
  cfblk16 : Outport  Port=2
  wires:
  cfblk4/1 -> cfblk16/1
  cfblk17/2(cfblk13) -> cfblk2/1
  cfblk10/1 -> cfblk17/Action
  cfblk10/2 -> cfblk18/Action
  cfblk11/1 -> cfblk19/Action
  cfblk11/2 -> cfblk20/Action
  cfblk12/1 -> cfblk21/Action
  cfblk12/2 -> cfblk22/Action
  cyemi_109/1 -> cfblk10/1
  cfblk25/1 -> cyemi_109/1
  cyemi_110/1 -> cfblk11/1
  cfblk26/1 -> cyemi_110/1
  cyemi_111/1 -> cfblk12/1
  cfblk20/2(cfblk10) -> cyemi_111/1
  cyemi_112/1 -> cfblk17/1(cfblk1)
  cfblk3/1 -> cyemi_112/1
  cyemi_113/1 -> cfblk17/2(cfblk11)
  cfblk7/1 -> cyemi_113/1
  cyemi_114/1 -> cfblk17/3(cfblk12)
  cfblk21/2(cfblk12) -> cyemi_114/1
  cyemi_127/1 -> cfblk18/1(cfblk1)
  cfblk22/3(cfblk13) -> cyemi_127/1
  cyemi_128/1 -> cfblk18/2(cfblk10)
  cfblk22/4(cfblk14) -> cyemi_128/1
  cyemi_138/1 -> cfblk19/1(cfblk1)
  cfblk27/1 -> cyemi_138/1
  cyemi_153/1 -> cfblk20/1(cfblk1)
  cfblk23/1 -> cyemi_153/1
  cyemi_154/1 -> cfblk20/2(cfblk8)
  cfblk1/1 -> cyemi_154/1
  cyemi_155/1 -> cfblk20/3(cfblk9)
  cfblk28/1 -> cyemi_155/1
  cyemi_164/1 -> cfblk21/1(cfblk1)
  cfblk13/1 -> cyemi_164/1
  cyemi_174/1 -> cfblk22/1(cfblk1)
  cfblk24/1 -> cyemi_174/1
  cyemi_175/1 -> cfblk22/2(cfblk11)
  cfblk19/3(cfblk14) -> cyemi_175/1
  cyemi_188/1 -> cfblk23/1
  cfblk19/1(cfblk2) -> cyemi_188/1
  cyemi_189/1 -> cfblk24/1
  cfblk5/1 -> cyemi_189/1
  cyemi_190/1 -> cfblk25/1
  cfblk18/1(cfblk2) -> cyemi_190/1
  cyemi_191/1 -> cfblk26/1
  cfblk20/1(cfblk2) -> cyemi_191/1
  cyemi_192/1 -> cfblk27/1
  cfblk21/1(cfblk2) -> cyemi_192/1
  cyemi_193/1 -> cfblk28/1
  cfblk9/1 -> cyemi_193/1
  cyemi_194/1 -> cfblk3/1
  cfblk22/1(cfblk2) -> cyemi_194/1
  cyemi_195/1 -> cfblk4/1
  cfblk8/1 -> cyemi_195/1
  cyemi_196/1 -> cfblk5/1
  cfblk6/1 -> cyemi_196/1
  cyemi_197/1 -> cfblk6/1
  cfblk17/1(cfblk2) -> cyemi_197/1
  cyemi_198/1 -> cfblk7/1
  cfblk22/2(cfblk12) -> cyemi_198/1
  cyemi_199/1 -> cfblk8/1
  cfblk19/2(cfblk13) -> cyemi_199/1
  cyemi_200/1 -> cfblk9/1
  cfblk21/3(cfblk13) -> cyemi_200/1

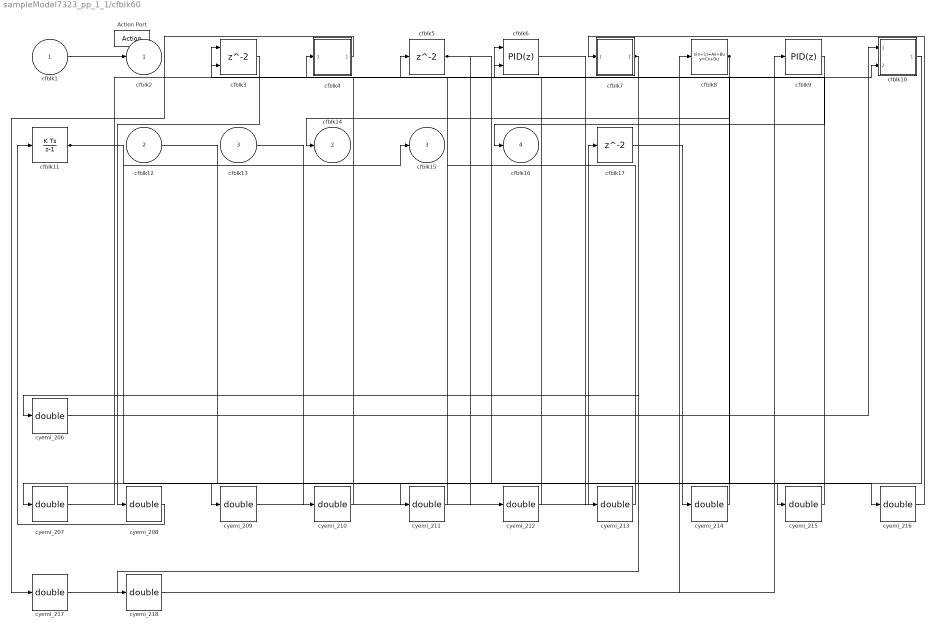
== system sampleModel7323_pp_1_1/cfblk60 ==
  cfblk1 : Inport
  cfblk12 : Inport  Port=2
  cfblk13 : Inport  Port=3
  Action Port : ActionPort  ActionType=else
  cfblk10 : Subsystem  TreatAsAtomicUnit=on
  cfblk11 : DiscreteIntegrator  SampleTime=-1  OutDataTypeStr=double  ICPrevOutput=DiscIntNeverNeededParam  ICPrevScaledInput=DiscIntNeverNeededParam
  cfblk17 : Delay
  cfblk3 : Delay  ShowEnablePort=on
      settings: InputPortMap=u0,e6
  cfblk4 : Subsystem  TreatAsAtomicUnit=on
  cfblk5 : Delay
  cfblk6 : simulink/Continuous/PID Controller (2DOF)  Controller=PID  TimeDomain=Discrete-time  SampleTime=-1  IntegratorMethod=Forward Euler  FilterMethod=Forward Euler  Form=Parallel  UseFilter=on  ControllerParametersSource=internal  P=1  I=1  D=0  N=100  b=1  c=1  InitialConditionSource=internal  InitialConditionForIntegrator=0  InitialConditionForFilter=0  ExternalReset=none  LimitOutput=off  UpperSaturationLimit=inf  LowerSaturationLimit=-inf  LinearizeAsGain=off  AntiWindupMode=none  Kb=1  TrackingMode=off  Kt=1  PParamMin=[]  PParamMax=[]  IParamMin=[]  IParamMax=[]  DParamMin=[]  DParamMax=[]  NParamMin=[]  NParamMax=[]  bParamMin=[]  bParamMax=[]  cParamMin=[]  cParamMax=[]  KbParamMin=[]  KbParamMax=[]  KtParamMin=[]  KtParamMax=[]  POutMin=[]  POutMax=[]  IOutMin=[]  IOutMax=[]  DOutMin=[]  DOutMax=[]  NOutMin=[]  NOutMax=[]  bOutMin=[]  bOutMax=[]  cOutMin=[]  cOutMax=[]  KbOutMin=[]  KbOutMax=[]  KtOutMin=[]  KtOutMax=[]  IntegratorOutMin=[]  IntegratorOutMax=[]  FilterOutMin=[]  FilterOutMax=[]  SumOutMin=[]  SumOutMax=[]  Sum1OutMin=[]  Sum1OutMax=[]  Sum2OutMin=[]  Sum2OutMax=[]  Sum3OutMin=[]  Sum3OutMax=[]  SumI1OutMin=[]  SumI1OutMax=[]  SumI2OutMin=[]  SumI2OutMax=[]  SumI3OutMin=[]  SumI3OutMax=[]  SumDOutMin=[]  SumDOutMax=[]  SaturationOutMin=[]  SaturationOutMax=[]  IntegratorContinuousStateAttributes=''  IntegratorStateMustResolveToSignalObject=off  IntegratorRTWStateStorageClass=Auto  FilterContinuousStateAttributes=''  FilterStateMustResolveToSignalObject=off  FilterRTWStateStorageClass=Auto  DifferentiatorICPrevScaledInput=0  DifferentiatorOutMin=[]  DifferentiatorOutMax=[]  FilterDiffOutCoefMin=[]  FilterDiffOutCoefMax=[]  SumDenOutMin=[]  SumDenOutMax=[]  SumNumOutMin=[]  SumNumOutMax=[]  ReciprocalOutMin=[]  ReciprocalOutMax=[]  DivideOutMin=[]  DivideOutMax=[]  TunerSelectOption=Transfer Function Based (PID Tuner App)
  cfblk7 : Subsystem  TreatAsAtomicUnit=on
  cfblk8 : DiscreteStateSpace  SampleTime=-1
  cfblk9 : simulink/Continuous/PID Controller  Controller=PID  TimeDomain=Discrete-time  SampleTime=-1  IntegratorMethod=Forward Euler  FilterMethod=Forward Euler  Form=Parallel  UseFilter=on  ControllerParametersSource=internal  P=1  I=1  D=0  N=100  InitialConditionSource=internal  InitialConditionForIntegrator=0  InitialConditionForFilter=0  ExternalReset=none  LimitOutput=off  UpperSaturationLimit=inf  LowerSaturationLimit=-inf  LinearizeAsGain=off  AntiWindupMode=none  Kb=1  TrackingMode=off  Kt=1  PParamMin=[]  PParamMax=[]  IParamMin=[]  IParamMax=[]  DParamMin=[]  DParamMax=[]  NParamMin=[]  NParamMax=[]  KbParamMin=[]  KbParamMax=[]  KtParamMin=[]  KtParamMax=[]  POutMin=[]  POutMax=[]  IOutMin=[]  IOutMax=[]  DOutMin=[]  DOutMax=[]  NOutMin=[]  NOutMax=[]  KbOutMin=[]  KbOutMax=[]  KtOutMin=[]  KtOutMax=[]  IntegratorOutMin=[]  IntegratorOutMax=[]  FilterOutMin=[]  FilterOutMax=[]  SumOutMin=[]  SumOutMax=[]  SumI1OutMin=[]  SumI1OutMax=[]  SumI2OutMin=[]  SumI2OutMax=[]  SumI3OutMin=[]  SumI3OutMax=[]  SumDOutMin=[]  SumDOutMax=[]  SaturationOutMin=[]  SaturationOutMax=[]  IntegratorContinuousStateAttributes=''  IntegratorStateMustResolveToSignalObject=off  IntegratorRTWStateStorageClass=Auto  FilterContinuousStateAttributes=''  FilterStateMustResolveToSignalObject=off  FilterRTWStateStorageClass=Auto  DifferentiatorICPrevScaledInput=0  DifferentiatorOutMin=[]  DifferentiatorOutMax=[]  FilterDiffOutCoefMin=[]  FilterDiffOutCoefMax=[]  SumDenOutMin=[]  SumDenOutMax=[]  SumNumOutMin=[]  SumNumOutMax=[]  ReciprocalOutMin=[]  ReciprocalOutMax=[]  DivideOutMin=[]  DivideOutMax=[]  TunerSelectOption=Transfer Function Based (PID Tuner App)
  cyemi_{206..218} (13 alike) : DataTypeConversion  OutDataTypeStr=double
  cfblk2 : Outport
  cfblk14 : Outport  Port=2
  cfblk15 : Outport  Port=3
  cfblk16 : Outport  Port=4
  wires:
  cfblk11/1 -> cfblk15/1, cyemi_215/1
  cfblk1/1 -> cfblk2/1
  cfblk9/1 -> cfblk16/1
  cfblk5/1 -> cyemi_212/1, cyemi_216/1
  cfblk8/1 -> cfblk14/1, cyemi_207/1
  cyemi_208/1 -> cfblk11/1
  cfblk3/1 -> cyemi_208/1
  cyemi_209/1 -> cfblk17/1
  cyemi_210/1 -> cfblk3/1
  cfblk13/1 -> cyemi_210/1
  cyemi_211/1 -> cfblk3/2
  cfblk12/1 -> cyemi_211/1
  cyemi_213/1 -> cfblk5/1
  cfblk6/1 -> cyemi_213/1
  cyemi_214/1 -> cfblk6/1
  cfblk17/1 -> cyemi_214/1
  cyemi_215/1 -> cfblk6/2
  cyemi_217/1 -> cfblk8/1
  cyemi_218/1 -> cfblk9/1
  cyemi_212/1 -> cfblk4/1(emi_100)
  cfblk4/1(emi_101) -> cyemi_217/1
  cyemi_206/1 -> cfblk10/1(emi_119)
  cyemi_207/1 -> cfblk10/2(emi_120)
  cfblk10/1(emi_121) -> cyemi_209/1
  cyemi_216/1 -> cfblk7/1(emi_127)
  cfblk7/1(emi_128) -> cyemi_206/1, cyemi_218/1

== system sampleModel7323_pp_1_1/cfblk63 ==
  emi_6 : Inport  Partition=on  PartitionDimension=1  PartitionWidth=1  PartitionOffset=0
  For Each : ForEach  DisableCoverage=on  IndexMode=One-based
  cfblk63 : Delay  SampleTime=1
  emi_7 : Outport  ConcatenationDimension=1
  wires:
  emi_6/1 -> cfblk63/1
  cfblk63/1 -> emi_7/1

== system sampleModel7323_pp_1_1/cfblk7 ==
  emi_15 : Inport  Partition=on  PartitionDimension=1  PartitionWidth=1  PartitionOffset=0
  For Each : ForEach  DisableCoverage=on  IndexMode=One-based
  cfblk7 : DiscreteStateSpace
  emi_16 : Outport  ConcatenationDimension=1
  wires:
  emi_15/1 -> cfblk7/1
  cfblk7/1 -> emi_16/1

== system sampleModel7323_pp_1_1/cfblk8 ==
  emi_85 : Inport  Partition=on  PartitionDimension=1  PartitionWidth=1  PartitionOffset=0
  For Each : ForEach  DisableCoverage=on  IndexMode=One-based
  cfblk8 : UnitDelay
  emi_86 : Outport  ConcatenationDimension=1
  wires:
  emi_85/1 -> cfblk8/1
  cfblk8/1 -> emi_86/1

== system sampleModel7323_pp_1_1/cfblk9 ==
  emi_107 : Inport  Partition=on  PartitionDimension=1  PartitionWidth=1  PartitionOffset=0
  For Each : ForEach  DisableCoverage=on  IndexMode=One-based
  cfblk9 : simulink/Continuous/PID Controller  Controller=PID  TimeDomain=Discrete-time  SampleTime=1  IntegratorMethod=Forward Euler  FilterMethod=Forward Euler  Form=Parallel  UseFilter=on  ControllerParametersSource=internal  P=1  I=1  D=0  N=100  InitialConditionSource=internal  InitialConditionForIntegrator=0  InitialConditionForFilter=0  ExternalReset=none  LimitOutput=off  UpperSaturationLimit=inf  LowerSaturationLimit=-inf  LinearizeAsGain=off  AntiWindupMode=none  Kb=1  TrackingMode=off  Kt=1  PParamMin=[]  PParamMax=[]  IParamMin=[]  IParamMax=[]  DParamMin=[]  DParamMax=[]  NParamMin=[]  NParamMax=[]  KbParamMin=[]  KbParamMax=[]  KtParamMin=[]  KtParamMax=[]  POutMin=[]  POutMax=[]  IOutMin=[]  IOutMax=[]  DOutMin=[]  DOutMax=[]  NOutMin=[]  NOutMax=[]  KbOutMin=[]  KbOutMax=[]  KtOutMin=[]  KtOutMax=[]  IntegratorOutMin=[]  IntegratorOutMax=[]  FilterOutMin=[]  FilterOutMax=[]  SumOutMin=[]  SumOutMax=[]  SumI1OutMin=[]  SumI1OutMax=[]  SumI2OutMin=[]  SumI2OutMax=[]  SumI3OutMin=[]  SumI3OutMax=[]  SumDOutMin=[]  SumDOutMax=[]  SaturationOutMin=[]  SaturationOutMax=[]  IntegratorContinuousStateAttributes=''  IntegratorStateMustResolveToSignalObject=off  IntegratorRTWStateStorageClass=Auto  FilterContinuousStateAttributes=''  FilterStateMustResolveToSignalObject=off  FilterRTWStateStorageClass=Auto  DifferentiatorICPrevScaledInput=0  DifferentiatorOutMin=[]  DifferentiatorOutMax=[]  FilterDiffOutCoefMin=[]  FilterDiffOutCoefMax=[]  SumDenOutMin=[]  SumDenOutMax=[]  SumNumOutMin=[]  SumNumOutMax=[]  ReciprocalOutMin=[]  ReciprocalOutMax=[]  DivideOutMin=[]  DivideOutMax=[]  TunerSelectOption=Transfer Function Based (PID Tuner App)
  emi_108 : Outport  ConcatenationDimension=1
  wires:
  emi_107/1 -> cfblk9/1
  cfblk9/1 -> emi_108/1

== system sampleModel7323_pp_1_1/cfblk20/cfblk20 ==
  emi_33 : Inport  Partition=on  PartitionDimension=1  PartitionWidth=1  PartitionOffset=0
  For Each : ForEach  DisableCoverage=on  IndexMode=One-based
  cfblk20 : simulink/Discrete/Transfer Fcn First Order  PoleZ=0.95  ICPrevOutput=0.0  DoSatur=off
      settings: SourceProductName=Simulink
  emi_34 : Outport  ConcatenationDimension=1
  wires:
  cfblk20/1 -> emi_34/1
  emi_33/1 -> cfblk20/1

== system sampleModel7323_pp_1_1/cfblk23/cfblk23 ==
  emi_60 : Inport  Partition=on  PartitionDimension=1  PartitionWidth=1  PartitionOffset=0
  emi_61 : Inport  Port=2  Partition=on  PartitionDimension=1  PartitionWidth=1  PartitionOffset=0
  For Each : ForEach  DisableCoverage=on  IndexMode=One-based
  cfblk23 : Delay  DelayLengthSource=Input port  SampleTime=1
      settings: InputPortMap=u0,p1
  emi_62 : Outport  ConcatenationDimension=1
  wires:
  cfblk23/1 -> emi_62/1
  emi_61/1 -> cfblk23/2
  emi_60/1 -> cfblk23/1

== system sampleModel7323_pp_1_1/cfblk49/cfblk49 ==
  For Each : ForEach  DisableCoverage=on  IndexMode=One-based
  cfblk49 : simulink/Sources/Counter Free-Running  NumBits=16  tsamp=1
  emi_4 : Outport  ConcatenationDimension=1
  wires:
  cfblk49/1 -> emi_4/1

== system sampleModel7323_pp_1_1/cfblk55/cfblk16 ==
  cfblk1 : Inport
  cfblk9 : Inport  Port=2
  cfblk10 : Inport  Port=3
  cfblk11 : Inport  Port=4
  Action Port : ActionPort  ActionType=then
  cfblk3 : simulink/Discrete/Transfer Fcn Real Zero  ZeroZ=0.75  ICPrevInput=0.0  DoSatur=off
      settings: SourceProductName=Simulink  SourceProductBaseCode=SL
  cfblk4 : simulink/Discrete/Tapped Delay  vinit=0.0  samptime=-1  NumDelays=1  DelayOrder=Oldest  includeCurrent=off
  cfblk5 : DiscreteZeroPole  Poles=[0 0.5]  Gain=1  SampleTime=-1
  cfblk6 : DiscreteFir
  cfblk7 : Delay  DelayLengthSource=Input port
      settings: InputPortMap=u0,p1
  cfblk8 : simulink/Discrete/Tapped Delay  vinit=0.0  samptime=-1  NumDelays=1  DelayOrder=Oldest  includeCurrent=off
  cyemi_{42..48} (7 alike) : DataTypeConversion  OutDataTypeStr=double
  cfblk2 : Outport
  cfblk12 : Outport  Port=2
  wires:
  cfblk4/1 -> cfblk2/1
  cfblk6/1 -> cfblk12/1
  cyemi_42/1 -> cfblk3/1
  cfblk10/1 -> cyemi_42/1
  cyemi_43/1 -> cfblk4/1
  cfblk5/1 -> cyemi_43/1
  cyemi_44/1 -> cfblk5/1
  cfblk9/1 -> cyemi_44/1
  cyemi_45/1 -> cfblk6/1
  cfblk7/1 -> cyemi_45/1
  cyemi_46/1 -> cfblk7/1
  cfblk1/1 -> cyemi_46/1
  cyemi_47/1 -> cfblk7/2
  cfblk11/1 -> cyemi_47/1
  cyemi_48/1 -> cfblk8/1
  cfblk3/1 -> cyemi_48/1

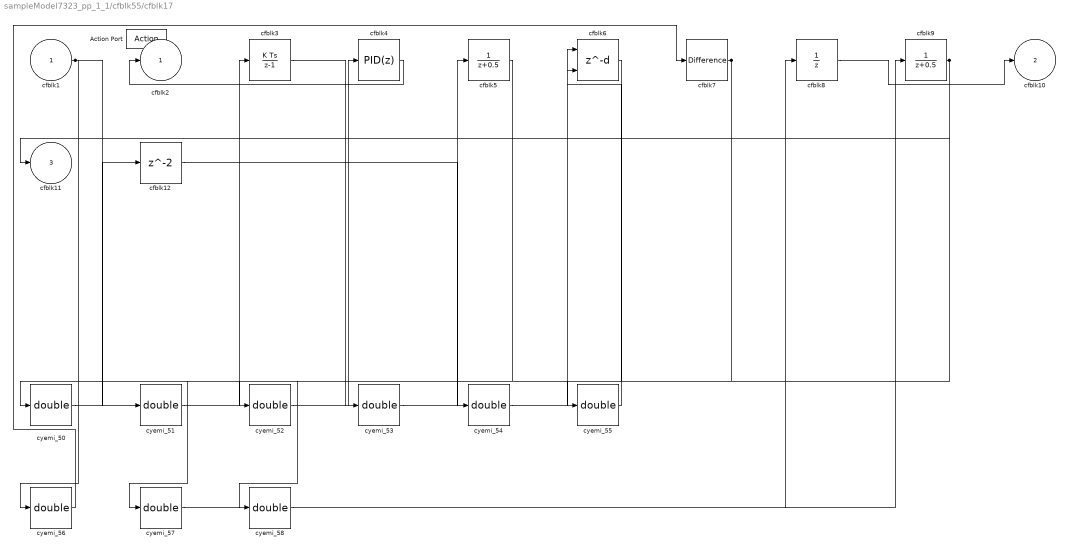
== system sampleModel7323_pp_1_1/cfblk55/cfblk17 ==
  cfblk1 : Inport
  Action Port : ActionPort  ActionType=else
  cfblk12 : Delay
  cfblk3 : DiscreteIntegrator  SampleTime=-1  OutDataTypeStr=double  ICPrevOutput=DiscIntNeverNeededParam  ICPrevScaledInput=DiscIntNeverNeededParam
  cfblk4 : simulink/Continuous/PID Controller  Controller=PID  TimeDomain=Discrete-time  SampleTime=-1  IntegratorMethod=Forward Euler  FilterMethod=Forward Euler  Form=Parallel  UseFilter=on  ControllerParametersSource=internal  P=1  I=1  D=0  N=100  InitialConditionSource=internal  InitialConditionForIntegrator=0  InitialConditionForFilter=0  ExternalReset=none  LimitOutput=off  UpperSaturationLimit=inf  LowerSaturationLimit=-inf  LinearizeAsGain=off  AntiWindupMode=none  Kb=1  TrackingMode=off  Kt=1  PParamMin=[]  PParamMax=[]  IParamMin=[]  IParamMax=[]  DParamMin=[]  DParamMax=[]  NParamMin=[]  NParamMax=[]  KbParamMin=[]  KbParamMax=[]  KtParamMin=[]  KtParamMax=[]  POutMin=[]  POutMax=[]  IOutMin=[]  IOutMax=[]  DOutMin=[]  DOutMax=[]  NOutMin=[]  NOutMax=[]  KbOutMin=[]  KbOutMax=[]  KtOutMin=[]  KtOutMax=[]  IntegratorOutMin=[]  IntegratorOutMax=[]  FilterOutMin=[]  FilterOutMax=[]  SumOutMin=[]  SumOutMax=[]  SumI1OutMin=[]  SumI1OutMax=[]  SumI2OutMin=[]  SumI2OutMax=[]  SumI3OutMin=[]  SumI3OutMax=[]  SumDOutMin=[]  SumDOutMax=[]  SaturationOutMin=[]  SaturationOutMax=[]  IntegratorContinuousStateAttributes=''  IntegratorStateMustResolveToSignalObject=off  IntegratorRTWStateStorageClass=Auto  FilterContinuousStateAttributes=''  FilterStateMustResolveToSignalObject=off  FilterRTWStateStorageClass=Auto  DifferentiatorICPrevScaledInput=0  DifferentiatorOutMin=[]  DifferentiatorOutMax=[]  FilterDiffOutCoefMin=[]  FilterDiffOutCoefMax=[]  SumDenOutMin=[]  SumDenOutMax=[]  SumNumOutMin=[]  SumNumOutMax=[]  ReciprocalOutMin=[]  ReciprocalOutMax=[]  DivideOutMin=[]  DivideOutMax=[]  TunerSelectOption=Transfer Function Based (PID Tuner App)
  cfblk5 : DiscreteTransferFcn
  cfblk6 : Delay  DelayLengthSource=Input port
      settings: InputPortMap=u0,p1
  cfblk7 : simulink/Discrete/Difference  ICPrevInput=0.0  OutMin=[]  OutMax=[]  OutDataTypeStr=double  OutputDataTypeScalingMode=double  OutDataType=fixdt(1, 16)  OutScaling=2^-10  DoSatur=off
  cfblk8 : UnitDelay  SampleTime=-1
  cfblk9 : DiscreteTransferFcn
  cyemi_{50..58} (9 alike) : DataTypeConversion  OutDataTypeStr=double
  cfblk2 : Outport
  cfblk10 : Outport  Port=2
  cfblk11 : Outport  Port=3
  wires:
  cfblk4/1 -> cfblk2/1
  cfblk8/1 -> cfblk10/1
  cfblk7/1 -> cyemi_52/1, cyemi_55/1
  cfblk1/1 -> cyemi_51/1, cyemi_56/1
  cfblk9/1 -> cfblk11/1, cyemi_50/1
  cyemi_50/1 -> cfblk12/1
  cyemi_51/1 -> cfblk3/1
  cyemi_52/1 -> cfblk4/1
  cyemi_53/1 -> cfblk5/1
  cfblk3/1 -> cyemi_53/1
  cyemi_54/1 -> cfblk6/1
  cfblk12/1 -> cyemi_54/1
  cyemi_55/1 -> cfblk6/2
  cyemi_56/1 -> cfblk7/1
  cyemi_57/1 -> cfblk8/1
  cfblk5/1 -> cyemi_57/1
  cyemi_58/1 -> cfblk9/1
  cfblk6/1 -> cyemi_58/1

== system sampleModel7323_pp_1_1/cfblk56/cfblk3 ==
  emi_110 : Inport  Partition=on  PartitionDimension=1  PartitionWidth=1  PartitionOffset=0
  For Each : ForEach  DisableCoverage=on  IndexMode=One-based
  cfblk3 : simulink/Discrete/Transfer Fcn First Order  PoleZ=0.95  ICPrevOutput=0.0  DoSatur=off
      settings: SourceProductName=Simulink
  emi_111 : Outport  ConcatenationDimension=1
  wires:
  emi_110/1 -> cfblk3/1
  cfblk3/1 -> emi_111/1

== system sampleModel7323_pp_1_1/cfblk56/cfblk5 ==
  emi_21 : Inport  Partition=on  PartitionDimension=1  PartitionWidth=1  PartitionOffset=0
  For Each : ForEach  DisableCoverage=on  IndexMode=One-based
  cfblk5 : DiscreteStateSpace  SampleTime=-1
  emi_22 : Outport  ConcatenationDimension=1
  wires:
  emi_21/1 -> cfblk5/1
  cfblk5/1 -> emi_22/1

== system sampleModel7323_pp_1_1/cfblk56/cfblk6 ==
  emi_1 : Inport  Partition=on  PartitionDimension=1  PartitionWidth=1  PartitionOffset=0
  For Each : ForEach  DisableCoverage=on  IndexMode=One-based
  cfblk6 : simulink/Discrete/Transfer Fcn First Order  PoleZ=0.95  ICPrevOutput=0.0  DoSatur=off
      settings: SourceProductName=Simulink
  emi_2 : Outport  ConcatenationDimension=1
  wires:
  emi_1/1 -> cfblk6/1
  cfblk6/1 -> emi_2/1

== system sampleModel7323_pp_1_1/cfblk57/cfblk10 ==
  emi_57 : Inport  Partition=on  PartitionDimension=1  PartitionWidth=1  PartitionOffset=0
  For Each : ForEach  DisableCoverage=on  IndexMode=One-based
  cfblk10 : Delay
  emi_58 : Outport  ConcatenationDimension=1
  wires:
  emi_57/1 -> cfblk10/1
  cfblk10/1 -> emi_58/1

== system sampleModel7323_pp_1_1/cfblk57/cfblk6 ==
  emi_24 : Inport  Partition=on  PartitionDimension=1  PartitionWidth=1  PartitionOffset=0
  For Each : ForEach  DisableCoverage=on  IndexMode=One-based
  cfblk6 : simulink/Discrete/Transfer Fcn Real Zero  ZeroZ=0.75  ICPrevInput=0.0  DoSatur=off
      settings: SourceProductName=Simulink  SourceProductBaseCode=SL
  emi_25 : Outport  ConcatenationDimension=1
  wires:
  emi_24/1 -> cfblk6/1
  cfblk6/1 -> emi_25/1

== system sampleModel7323_pp_1_1/cfblk57/cfblk7 ==
  emi_97 : Inport  Partition=on  PartitionDimension=1  PartitionWidth=1  PartitionOffset=0
  For Each : ForEach  DisableCoverage=on  IndexMode=One-based
  cfblk7 : simulink/Continuous/PID Controller  Controller=PID  TimeDomain=Discrete-time  SampleTime=-1  IntegratorMethod=Forward Euler  FilterMethod=Forward Euler  Form=Parallel  UseFilter=on  ControllerParametersSource=internal  P=1  I=1  D=0  N=100  InitialConditionSource=internal  InitialConditionForIntegrator=0  InitialConditionForFilter=0  ExternalReset=none  LimitOutput=off  UpperSaturationLimit=inf  LowerSaturationLimit=-inf  LinearizeAsGain=off  AntiWindupMode=none  Kb=1  TrackingMode=off  Kt=1  PParamMin=[]  PParamMax=[]  IParamMin=[]  IParamMax=[]  DParamMin=[]  DParamMax=[]  NParamMin=[]  NParamMax=[]  KbParamMin=[]  KbParamMax=[]  KtParamMin=[]  KtParamMax=[]  POutMin=[]  POutMax=[]  IOutMin=[]  IOutMax=[]  DOutMin=[]  DOutMax=[]  NOutMin=[]  NOutMax=[]  KbOutMin=[]  KbOutMax=[]  KtOutMin=[]  KtOutMax=[]  IntegratorOutMin=[]  IntegratorOutMax=[]  FilterOutMin=[]  FilterOutMax=[]  SumOutMin=[]  SumOutMax=[]  SumI1OutMin=[]  SumI1OutMax=[]  SumI2OutMin=[]  SumI2OutMax=[]  SumI3OutMin=[]  SumI3OutMax=[]  SumDOutMin=[]  SumDOutMax=[]  SaturationOutMin=[]  SaturationOutMax=[]  IntegratorContinuousStateAttributes=''  IntegratorStateMustResolveToSignalObject=off  IntegratorRTWStateStorageClass=Auto  FilterContinuousStateAttributes=''  FilterStateMustResolveToSignalObject=off  FilterRTWStateStorageClass=Auto  DifferentiatorICPrevScaledInput=0  DifferentiatorOutMin=[]  DifferentiatorOutMax=[]  FilterDiffOutCoefMin=[]  FilterDiffOutCoefMax=[]  SumDenOutMin=[]  SumDenOutMax=[]  SumNumOutMin=[]  SumNumOutMax=[]  ReciprocalOutMin=[]  ReciprocalOutMax=[]  DivideOutMin=[]  DivideOutMax=[]  TunerSelectOption=Transfer Function Based (PID Tuner App)
  emi_98 : Outport  ConcatenationDimension=1
  wires:
  emi_97/1 -> cfblk7/1
  cfblk7/1 -> emi_98/1

== system sampleModel7323_pp_1_1/cfblk57/cfblk9 ==
  emi_42 : Inport  Partition=on  PartitionDimension=1  PartitionWidth=1  PartitionOffset=0
  For Each : ForEach  DisableCoverage=on  IndexMode=One-based
  cfblk9 : DiscreteTransferFcn
  emi_43 : Outport  ConcatenationDimension=1
  wires:
  emi_42/1 -> cfblk9/1
  cfblk9/1 -> emi_43/1

== system sampleModel7323_pp_1_1/cfblk58/cfblk10 ==
  emi_12 : Inport  Partition=on  PartitionDimension=1  PartitionWidth=1  PartitionOffset=0
  For Each : ForEach  DisableCoverage=on  IndexMode=One-based
  cfblk10 : DiscreteFilter
  emi_13 : Outport  ConcatenationDimension=1
  wires:
  emi_12/1 -> cfblk10/1
  cfblk10/1 -> emi_13/1
